simulink model "Vf_control"  (R2024a)
settings: Solver=ode23s  StartTime=0.0  StopTime=5  MaxStep=0.00001  RelTol=1e-3
libraries: dspfdesign x6, spsMosfetLib x6, spsVoltageMeasurementLib x3, simulink x1, autolibpmsmexterior x1, spsDCVoltageSourceLib x1, sps_lib x1
settings Model: Creator=hzn  LastModifiedBy=hzn

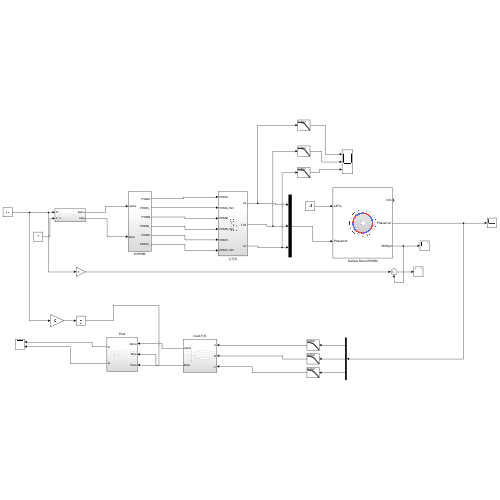
[thumbnail: Simulink's stored preview of the top-level diagram]
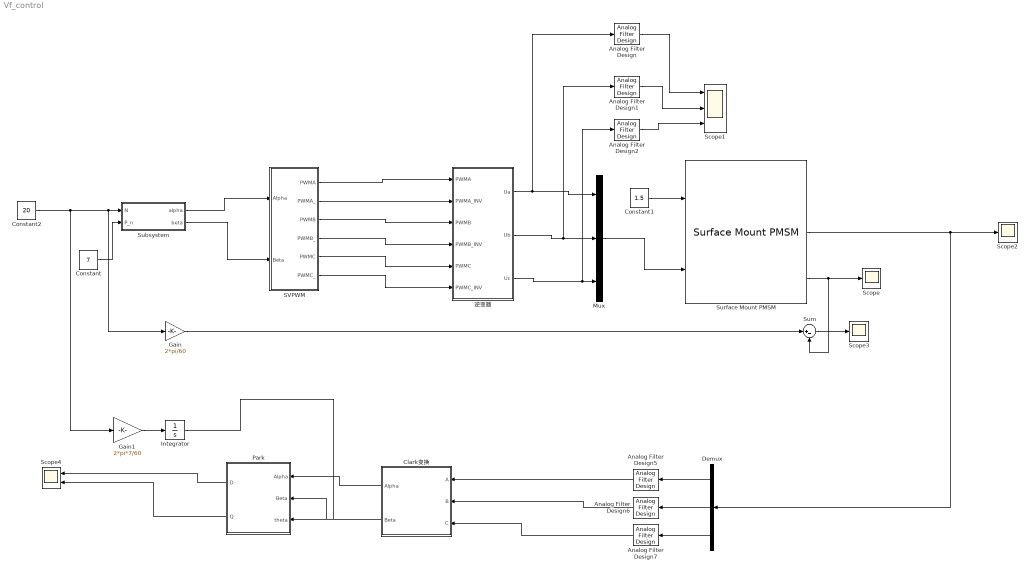
== system Vf_control ==
  Analog Filter Design : dspfdesign/Analog Filter Design  method=Butterworth  filttype=Lowpass  N=2  Wlo=30  Whi=80  Rp=2  Rs=40
  Analog Filter Design1 : dspfdesign/Analog Filter Design  method=Butterworth  filttype=Lowpass  N=2  Wlo=30  Whi=80  Rp=2  Rs=40
  Analog Filter Design2 : dspfdesign/Analog Filter Design  method=Butterworth  filttype=Lowpass  N=2  Wlo=30  Whi=80  Rp=2  Rs=40
  Analog Filter Design5 : dspfdesign/Analog Filter Design  method=Butterworth  filttype=Lowpass  N=1  Wlo=10  Whi=80  Rp=2  Rs=40
  Analog Filter Design6 : dspfdesign/Analog Filter Design  method=Butterworth  filttype=Lowpass  N=1  Wlo=10  Whi=80  Rp=2  Rs=40
  Analog Filter Design7 : dspfdesign/Analog Filter Design  method=Butterworth  filttype=Lowpass  N=1  Wlo=10  Whi=80  Rp=2  Rs=40
  Clark变换 : Subsystem
  Constant : Constant  Value=7
  Constant1 : Constant  Value=1.5
  Constant2 : Constant  Value=20
  Demux : Demux  Outputs=3
  Gain : Gain  Gain=2*pi/60
  Gain1 : Gain  Gain=2*pi*7/60
  Integrator : Integrator
  Mux : Mux  Inputs=3
  Park : Subsystem
  SVPWM : Subsystem
  Scope : Scope
  Scope1 : Scope  NumInputPorts=3
  Scope2 : Scope
  Scope3 : Scope
  Scope4 : Scope  NumInputPorts=2
  Subsystem : Subsystem
  Sum : Sum  Inputs=|+-
  Surface Mount PMSM : autolibpmsmexterior/Surface Mount PMSM  port_config=Torque  sim_type=Continuous  Ts=0.001  FilePath=E:\Sandbox\Bauto\Work\surfacepmsm_motordata.m  P=7  Rs=0.12  Ldq_=3.752e-4  KConstText=Permanent flux linkage constant (lambda_pm):  lambda_pm=0.0194  Ke=159.9771  Kt=1.323  mechanical=[0.0027, 4.924e-4, 0]  idq0=[0 0]  theta_init=0  omega_init=0  KConst=0.0194  lambda_pm_calc=0.0194  RefBlkName='autolibpmsmexterior/Surface Mount PMSM'  aMode=1  Ldq="[0.0003752   0.0003752]"
      settings: LibrarySourceBlock=autolibemachines/Surface Mount PMSM
  逆变器 : Subsystem
  wires:
  SVPWM/4(PWMB_) -> 逆变器/4(PWMB_INV)
  SVPWM/6(PWMC_) -> 逆变器/6(PWMC_INV)
  SVPWM/5(PWMC) -> 逆变器/5(PWMC)
  SVPWM/1(PWMA) -> 逆变器/1(PWMA)
  SVPWM/3(PWMB) -> 逆变器/3(PWMB)
  SVPWM/2(PWMA_) -> 逆变器/2(PWMA_INV)
  Mux/1 -> Surface Mount PMSM/2
  Constant1/1 -> Surface Mount PMSM/1
  Constant/1 -> Subsystem/2(P_n)
  逆变器/1(Ua) -> Analog Filter Design/1, Mux/1
  Analog Filter Design2/1 -> Scope1/3
  Analog Filter Design/1 -> Scope1/1
  逆变器/3(Uc) -> Analog Filter Design2/1, Mux/3
  逆变器/2(Ub) -> Analog Filter Design1/1, Mux/2
  Analog Filter Design1/1 -> Scope1/2
  Subsystem/1(alpha) -> SVPWM/1(Alpha)
  Subsystem/2(beta) -> SVPWM/2(Beta)
  Surface Mount PMSM/3 -> Sum/2, Scope/1
  Gain/1 -> Sum/1
  Sum/1 -> Scope3/1
  Analog Filter Design5/1 -> Clark变换/1(A)
  Analog Filter Design7/1 -> Clark变换/3(C)
  Park/2(Q) -> Scope4/2
  Analog Filter Design6/1 -> Clark变换/2(B)
  Surface Mount PMSM/2 -> Demux/1, Scope2/1
  Demux/2 -> Analog Filter Design6/1
  Park/1(D) -> Scope4/1
  Clark变换/1(Alpha) -> Park/1(Alpha)
  Demux/3 -> Analog Filter Design7/1
  Clark变换/2(Beta) -> Park/2(Beta)
  Demux/1 -> Analog Filter Design5/1
  Constant2/1 -> Gain1/1, Gain/1, Subsystem/1(N)
  Integrator/1 -> Park/3(theta)
  Gain1/1 -> Integrator/1

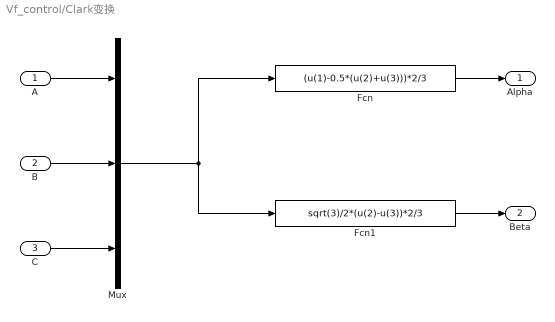
== system Vf_control/Clark变换 ==
  A : Inport
  B : Inport  Port=2
  C : Inport  Port=3
  Fcn : Fcn  Expr=(u(1)-0.5*(u(2)+u(3)))*2/3
  Fcn1 : Fcn  Expr=sqrt(3)/2*(u(2)-u(3))*2/3
  Mux : Mux  Inputs=3
  Alpha : Outport
  Beta : Outport  Port=2
  wires:
  B/1 -> Mux/2
  A/1 -> Mux/1
  C/1 -> Mux/3
  Mux/1 -> Fcn1/1, Fcn/1
  Fcn/1 -> Alpha/1
  Fcn1/1 -> Beta/1

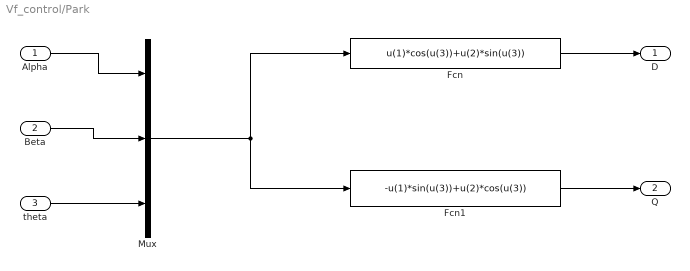
== system Vf_control/Park ==
  Alpha : Inport
  Beta : Inport  Port=2
  theta : Inport  Port=3
  Fcn : Fcn  Expr=u(1)*cos(u(3))+u(2)*sin(u(3))
  Fcn1 : Fcn  Expr=-u(1)*sin(u(3))+u(2)*cos(u(3))
  Mux : Mux  Inputs=3
  D : Outport
  Q : Outport  Port=2
  wires:
  Alpha/1 -> Mux/1
  Beta/1 -> Mux/2
  theta/1 -> Mux/3
  Mux/1 -> Fcn/1, Fcn1/1
  Fcn/1 -> D/1
  Fcn1/1 -> Q/1

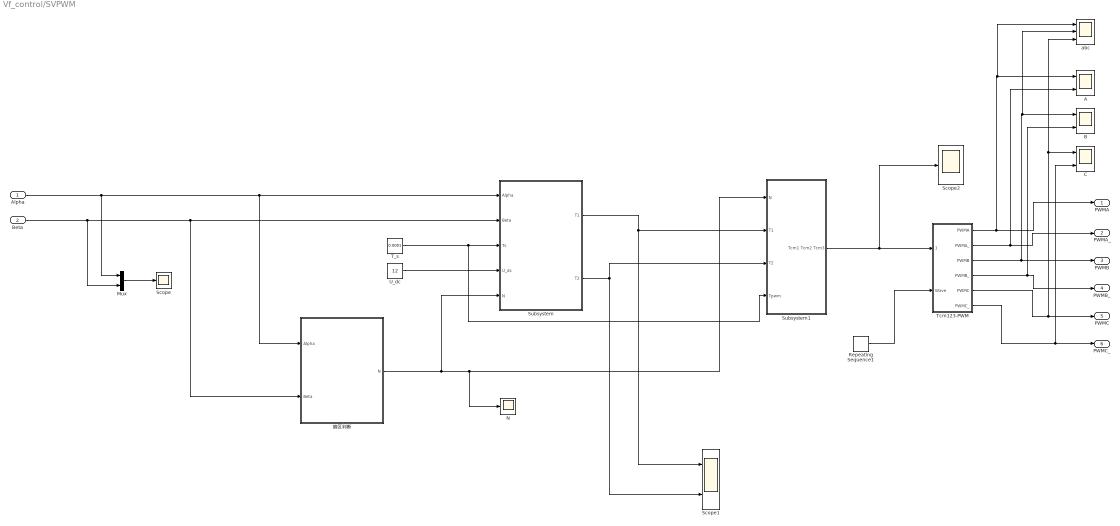
== system Vf_control/SVPWM ==
  Alpha : Inport
  Beta : Inport  Port=2
  A : Scope  NumInputPorts=2
  B : Scope  NumInputPorts=2
  C : Scope  NumInputPorts=2
  Mux : Mux  Inputs=2
  N : Scope
  Repeating Sequence1 : simulink/Sources/Repeating Sequence  rep_seq_t=[0 0.0001/2 0.0001]  rep_seq_y=[0 0.0001/2 0]
  Scope : Scope
  Scope1 : Scope  NumInputPorts=2
  Scope2 : Scope
  Subsystem : Subsystem
  Subsystem1 : Subsystem
  T_s : Constant  Value=0.0001
  Tcm123-PWM : Subsystem
  U_dc : Constant  Value=12
  abc : Scope  NumInputPorts=3
  扇区判断 : Subsystem
  PWMA : Outport
  PWMA_ : Outport  Port=2
  PWMB : Outport  Port=3
  PWMB_ : Outport  Port=4
  PWMC : Outport  Port=5
  PWMC_ : Outport  Port=6
  wires:
  U_dc/1 -> Subsystem/4(U_dc)
  Subsystem/1(T1) -> Scope1/1, Subsystem1/2(T1)
  Subsystem/2(T2) -> Scope1/2, Subsystem1/3(T2)
  Alpha/1 -> Mux/1, Subsystem/1(Alpha), 扇区判断/1(Alpha)
  Mux/1 -> Scope/1
  Beta/1 -> Mux/2, Subsystem/2(Beta), 扇区判断/2(Beta)
  扇区判断/1(N) -> Subsystem/5(N), N/1, Subsystem1/1(N)
  T_s/1 -> Subsystem1/4(Tpwm), Subsystem/3(Ts)
  Subsystem1/1(Tcm1 Tcm2 Tcm3) -> Scope2/1, Tcm123-PWM/1(Tcm123)
  Repeating Sequence1/1 -> Tcm123-PWM/2(Wave)
  Tcm123-PWM/1(PWMA) -> abc/1, A/1, PWMA/1
  Tcm123-PWM/2(PWMA_) -> A/2, PWMA_/1
  Tcm123-PWM/3(PWMB) -> abc/2, B/1, PWMB/1
  Tcm123-PWM/4(PWMB_) -> B/2, PWMB_/1
  Tcm123-PWM/5(PWMC) -> abc/3, C/1, PWMC/1
  Tcm123-PWM/6(PWMC_) -> C/2, PWMC_/1

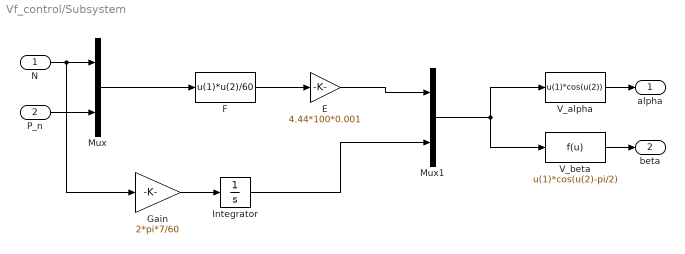
== system Vf_control/Subsystem ==
  N : Inport
  P_n : Inport  Port=2
  E : Gain  Gain=4.44*100*0.001
  F : Fcn  Expr=u(1)*u(2)/60
  Gain : Gain  Gain=2*pi*7/60
  Integrator : Integrator
  Mux : Mux  Inputs=2
  Mux1 : Mux  Inputs=2
  V_alpha : Fcn  Expr=u(1)*cos(u(2))
  V_beta : Fcn  Expr=u(1)*cos(u(2)-pi/2)
  alpha : Outport
  beta : Outport  Port=2
  wires:
  N/1 -> Gain/1, Mux/1
  P_n/1 -> Mux/2
  Mux/1 -> F/1
  F/1 -> E/1
  E/1 -> Mux1/1
  Gain/1 -> Integrator/1
  Integrator/1 -> Mux1/2
  Mux1/1 -> V_beta/1, V_alpha/1
  V_beta/1 -> beta/1
  V_alpha/1 -> alpha/1

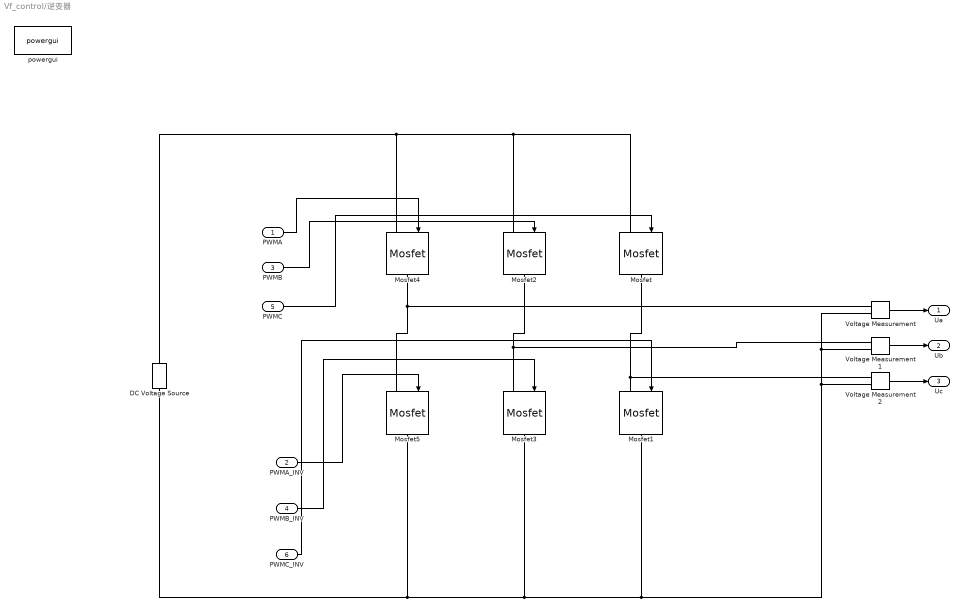
== system Vf_control/逆变器 ==
  PWMA : Inport
  PWMA_INV : Inport  Port=2
  PWMB : Inport  Port=3
  PWMB_INV : Inport  Port=4
  PWMC : Inport  Port=5
  PWMC_INV : Inport  Port=6
  DC Voltage Source : spsDCVoltageSourceLib/DC Voltage Source  Amplitude=12  Measurements=Voltage
  Mosfet{,1..5} (6 alike) : spsMosfetLib/Mosfet  Ron=0.1  Lon=0  Rd=0.01  Vfd=0  IC=0  Rs=1e5  Cs=inf  Measurements=off
  Voltage Measurement : spsVoltageMeasurementLib/Voltage Measurement  PhasorSimulation=off  OutputType=Complex  PSBequivalent=0
  Voltage Measurement1 : spsVoltageMeasurementLib/Voltage Measurement  PhasorSimulation=off  OutputType=Complex  PSBequivalent=0
  Voltage Measurement2 : spsVoltageMeasurementLib/Voltage Measurement  PhasorSimulation=off  OutputType=Complex  PSBequivalent=0
  powergui : sps_lib/powergui  Priority=1  SimulationMode=Continuous  SampleTime=50e-6  frequency=60  Iterations=50  frequencyindice=0  Pbase=100e6  ErrMax=1e-4  UnitsV=kV  UnitsW=MW  buscounter=0  FunctionMessages=off  echomessages=off  EnableUseOfTLC=off  CurrentSourceSwitches=off  DisableSnubberDevices=off  DisableRonSwitches=off  DisableVfSwitches=off  DisplayEquations=off  AutomaticDiscreteSolvers=off  SolverType=Tustin/Backward Euler (TBE)  Interpol=off  ExternalGateDelay=off  methode=off  Ts=100  x0status=blocks  SPID=on  SwTol=0  HookPort=off  NonlinearTolerance=1e-4  nMaxIteration=100  ContinueOnMaxIteration=off  RestoreLinks=warning  ResistiveCurrentMeasurement=off  Frange=[0:2:500]  Ylog=off  Xlog=on  ShowGrid=off  save=off  variable=ZData  structure=0  ZoomFFT=off  StartTime=0.0  cycles=1  DisplayStyle=1  fundamental=60  FreqAxis=off  MaxFrequency=1000  frequencyindicesteady=1  RmsSteady=1  display=off
  Ua : Outport
  Ub : Outport  Port=2
  Uc : Outport  Port=3
  wires:
  Voltage Measurement/1 -> Ua/1
  Voltage Measurement1/1 -> Ub/1
  Voltage Measurement2/1 -> Uc/1
  PWMC/1 -> Mosfet/1
  PWMB/1 -> Mosfet2/1
  PWMA/1 -> Mosfet4/1
  PWMA_INV/1 -> Mosfet5/1
  PWMB_INV/1 -> Mosfet3/1
  PWMC_INV/1 -> Mosfet1/1
  connections:
  Voltage Measurement/LConn2 -- Voltage Measurement1/LConn2 -- Mosfet1/RConn1 -- Mosfet3/RConn1 -- Mosfet5/RConn1 -- DC Voltage Source/LConn1 -- Voltage Measurement2/LConn2
  DC Voltage Source/RConn1 -- Mosfet4/LConn1 -- Mosfet2/LConn1 -- Mosfet/LConn1
  Mosfet4/RConn1 -- Voltage Measurement/LConn1 -- Mosfet5/LConn1
  Mosfet2/RConn1 -- Voltage Measurement1/LConn1 -- Mosfet3/LConn1
  Mosfet/RConn1 -- Voltage Measurement2/LConn1 -- Mosfet1/LConn1

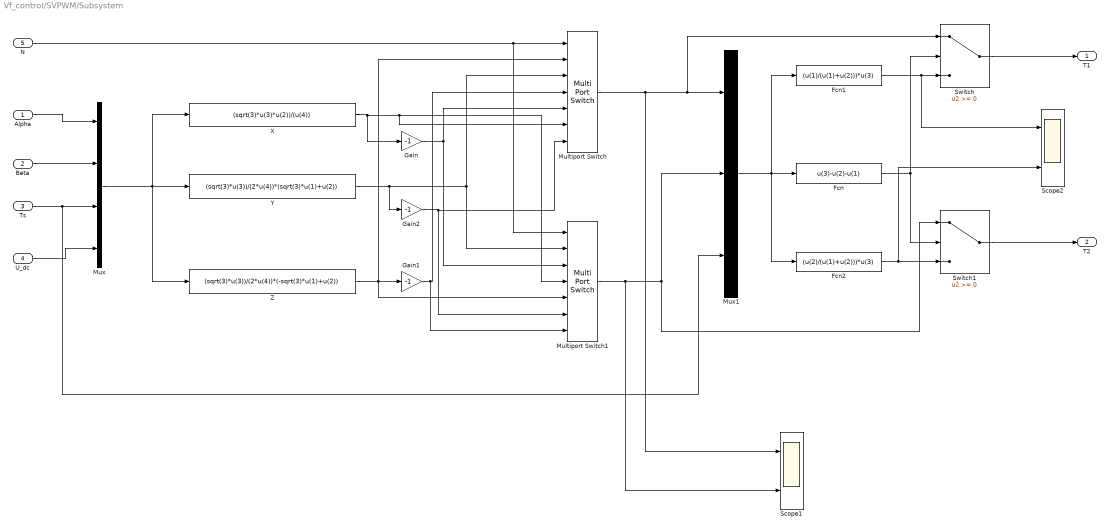
== system Vf_control/SVPWM/Subsystem ==
  Alpha : Inport
  Beta : Inport  Port=2
  Ts : Inport  Port=3
  U_dc : Inport  Port=4
  N : Inport  Port=5
  Fcn : Fcn  Expr=u(3)-u(2)-u(1)
  Fcn1 : Fcn  Expr=(u(1)/(u(1)+u(2)))*u(3)
  Fcn2 : Fcn  Expr=(u(2)/(u(1)+u(2)))*u(3)
  Gain : Gain  Gain=-1
  Gain1 : Gain  Gain=-1
  Gain2 : Gain  Gain=-1
  Multiport Switch : MultiPortSwitch  Inputs=6  SaturateOnIntegerOverflow=off  InputSameDT=off
  Multiport Switch1 : MultiPortSwitch  Inputs=6  SaturateOnIntegerOverflow=off  InputSameDT=off
  Mux : Mux
  Mux1 : Mux  Inputs=3
  Scope1 : Scope  NumInputPorts=2
  Scope2 : Scope  NumInputPorts=2
  Switch : Switch  SaturateOnIntegerOverflow=off  InputSameDT=off
  Switch1 : Switch  SaturateOnIntegerOverflow=off  InputSameDT=off
  X : Fcn  Expr=(sqrt(3)*u(3)*u(2))/(u(4))
  Y : Fcn  Expr=(sqrt(3)*u(3))/(2*u(4))*(sqrt(3)*u(1)+u(2))
  Z : Fcn  Expr=(sqrt(3)*u(3))/(2*u(4))*(-sqrt(3)*u(1)+u(2))
  T1 : Outport
  T2 : Outport  Port=2
  wires:
  Alpha/1 -> Mux/1
  Beta/1 -> Mux/2
  U_dc/1 -> Mux/4
  Mux/1 -> X/1, Z/1, Y/1
  Y/1 -> Gain2/1, Multiport Switch1/2, Multiport Switch/3
  Z/1 -> Multiport Switch1/5, Gain1/1, Multiport Switch/2
  X/1 -> Multiport Switch/6, Multiport Switch1/4, Gain/1
  N/1 -> Multiport Switch1/1, Multiport Switch/1
  Gain/1 -> Multiport Switch1/3, Multiport Switch/5
  Gain1/1 -> Multiport Switch1/7, Multiport Switch/4
  Gain2/1 -> Multiport Switch1/6, Multiport Switch/7
  Multiport Switch/1 -> Scope1/1, Switch/1, Mux1/1
  Ts/1 -> Mux1/3, Mux/3
  Mux1/1 -> Fcn2/1, Fcn1/1, Fcn/1
  Fcn1/1 -> Scope2/1, Switch/3
  Fcn/1 -> Switch/2, Switch1/2
  Multiport Switch1/1 -> Scope1/2, Mux1/2, Switch1/1
  Fcn2/1 -> Scope2/2, Switch1/3
  Switch/1 -> T1/1
  Switch1/1 -> T2/1

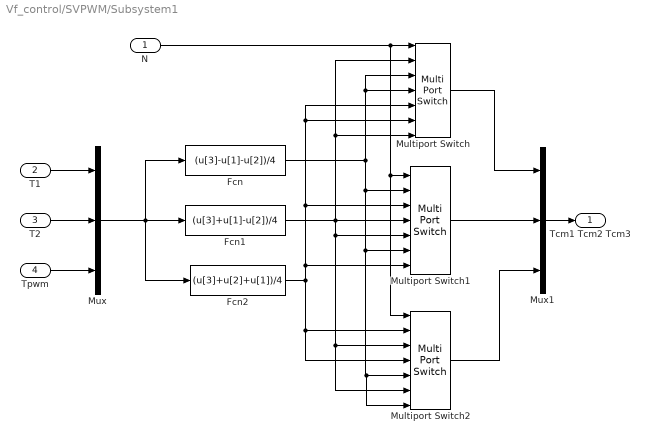
== system Vf_control/SVPWM/Subsystem1 ==
  N : Inport
  T1 : Inport  Port=2
  T2 : Inport  Port=3
  Tpwm : Inport  Port=4
  Fcn : Fcn  Expr=(u[3]-u[1]-u[2])/4
  Fcn1 : Fcn  Expr=(u[3]+u[1]-u[2])/4
  Fcn2 : Fcn  Expr=(u[3]+u[2]+u[1])/4
  Multiport Switch : MultiPortSwitch  Inputs=6  SaturateOnIntegerOverflow=off  InputSameDT=off
  Multiport Switch1 : MultiPortSwitch  Inputs=6  SaturateOnIntegerOverflow=off  InputSameDT=off
  Multiport Switch2 : MultiPortSwitch  Inputs=6  SaturateOnIntegerOverflow=off  InputSameDT=off
  Mux : Mux  Inputs=3
  Mux1 : Mux  Inputs=3
  Tcm1 Tcm2 Tcm3 : Outport
  wires:
  Fcn/1 -> Multiport Switch/3, Multiport Switch/4, Multiport Switch1/6, Multiport Switch2/5, Multiport Switch2/7, Multiport Switch1/2
  Mux/1 -> Fcn2/1, Fcn/1, Fcn1/1
  Multiport Switch/1 -> Mux1/1
  Multiport Switch2/1 -> Mux1/3
  Multiport Switch1/1 -> Mux1/2
  Mux1/1 -> Tcm1 Tcm2 Tcm3/1
  T2/1 -> Mux/2
  N/1 -> Multiport Switch2/1, Multiport Switch1/1, Multiport Switch/1
  Fcn2/1 -> Multiport Switch/5, Multiport Switch/6, Multiport Switch1/3, Multiport Switch1/7, Multiport Switch2/2, Multiport Switch2/4
  Tpwm/1 -> Mux/3
  Fcn1/1 -> Multiport Switch1/5, Multiport Switch2/3, Multiport Switch2/6, Multiport Switch1/4, Multiport Switch/7, Multiport Switch/2
  T1/1 -> Mux/1

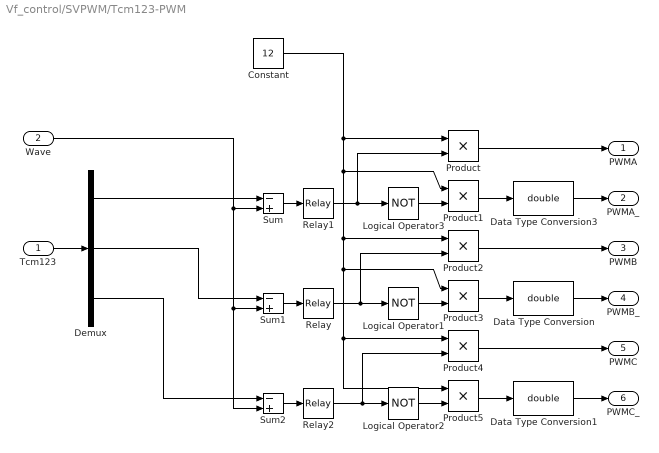
== system Vf_control/SVPWM/Tcm123-PWM ==
  Tcm123 : Inport
  Wave : Inport  Port=2
  Constant : Constant  Value=12
  Data Type Conversion : DataTypeConversion  OutDataTypeStr=double  SaturateOnIntegerOverflow=off  RndMeth=Floor
  Data Type Conversion1 : DataTypeConversion  OutDataTypeStr=double  SaturateOnIntegerOverflow=off  RndMeth=Floor
  Data Type Conversion3 : DataTypeConversion  OutDataTypeStr=double  SaturateOnIntegerOverflow=off  RndMeth=Floor
  Demux : Demux  Outputs=3
  Logical Operator1 : Logic  Operator=NOT  AllPortsSameDT=off  OutDataTypeStr=boolean
  Logical Operator2 : Logic  Operator=NOT  AllPortsSameDT=off  OutDataTypeStr=boolean
  Logical Operator3 : Logic  Operator=NOT  AllPortsSameDT=off  OutDataTypeStr=boolean
  Product{,1..5} (6 alike) : Product
  Relay : Relay  OffSwitchValue=-eps
  Relay1 : Relay  OffSwitchValue=-eps
  Relay2 : Relay  OffSwitchValue=-eps
  Sum : Sum  Inputs=-+  SaturateOnIntegerOverflow=on
  Sum1 : Sum  Inputs=-+  SaturateOnIntegerOverflow=on
  Sum2 : Sum  Inputs=-+  SaturateOnIntegerOverflow=on
  PWMA : Outport
  PWMA_ : Outport  Port=2
  PWMB : Outport  Port=3
  PWMB_ : Outport  Port=4
  PWMC : Outport  Port=5
  PWMC_ : Outport  Port=6
  wires:
  Tcm123/1 -> Demux/1
  Demux/3 -> Sum2/1
  Demux/2 -> Sum1/1
  Demux/1 -> Sum/1
  Wave/1 -> Sum1/2, Sum2/2, Sum/2
  Sum/1 -> Relay1/1
  Sum2/1 -> Relay2/1
  Sum1/1 -> Relay/1
  Relay1/1 -> Product/2, Logical Operator3/1
  Relay2/1 -> Product4/2, Logical Operator2/1
  Relay/1 -> Product2/2, Logical Operator1/1
  Logical Operator3/1 -> Product1/2
  Logical Operator1/1 -> Product3/2
  Logical Operator2/1 -> Product5/2
  Data Type Conversion3/1 -> PWMA_/1
  Data Type Conversion/1 -> PWMB_/1
  Data Type Conversion1/1 -> PWMC_/1
  Product1/1 -> Data Type Conversion3/1
  Product3/1 -> Data Type Conversion/1
  Product5/1 -> Data Type Conversion1/1
  Product/1 -> PWMA/1
  Product2/1 -> PWMB/1
  Product4/1 -> PWMC/1
  Constant/1 -> Product/1, Product1/1, Product2/1, Product4/1, Product5/1, Product3/1

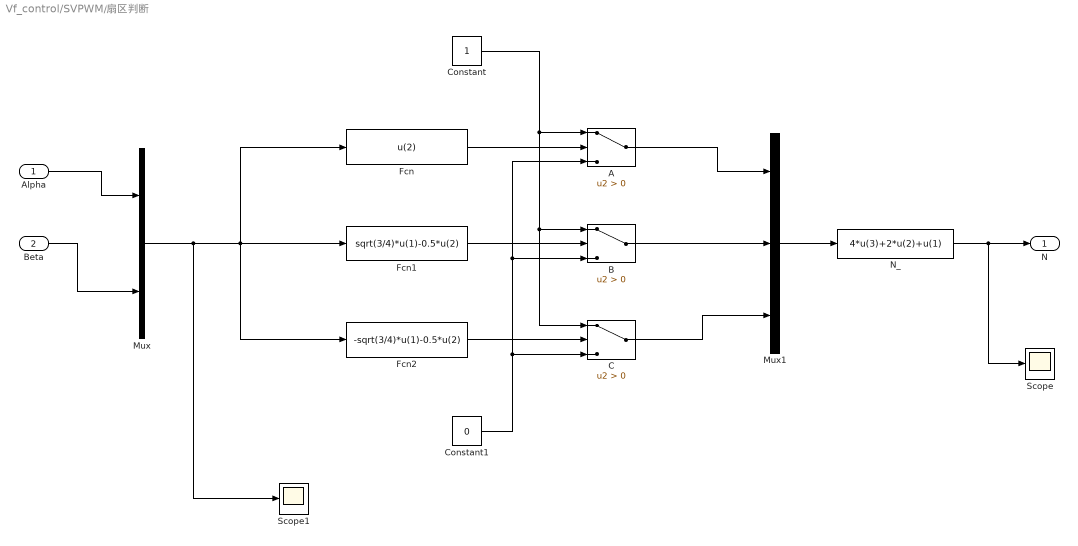
== system Vf_control/SVPWM/扇区判断 ==
  Alpha : Inport
  Beta : Inport  Port=2
  A : Switch  Criteria=u2 > Threshold  SaturateOnIntegerOverflow=off  InputSameDT=off
  B : Switch  Criteria=u2 > Threshold  SaturateOnIntegerOverflow=off  InputSameDT=off
  C : Switch  Criteria=u2 > Threshold  SaturateOnIntegerOverflow=off  InputSameDT=off
  Constant : Constant
  Constant1 : Constant  Value=0
  Fcn : Fcn  Expr=u(2)
  Fcn1 : Fcn  Expr=sqrt(3/4)*u(1)-0.5*u(2)
  Fcn2 : Fcn  Expr=-sqrt(3/4)*u(1)-0.5*u(2)
  Mux : Mux  Inputs=2
  Mux1 : Mux  Inputs=3
  N_ : Fcn  Expr=4*u(3)+2*u(2)+u(1)
  Scope : Scope
  Scope1 : Scope
  N : Outport
  wires:
  Alpha/1 -> Mux/1
  Beta/1 -> Mux/2
  Mux/1 -> Scope1/1, Fcn2/1, Fcn1/1, Fcn/1
  Fcn/1 -> A/2
  Fcn1/1 -> B/2
  Fcn2/1 -> C/2
  Constant/1 -> C/1, B/1, A/1
  Constant1/1 -> C/3, A/3, B/3
  A/1 -> Mux1/1
  B/1 -> Mux1/2
  C/1 -> Mux1/3
  Mux1/1 -> N_/1
  N_/1 -> Scope/1, N/1
